simulink model "demonstrator"  (R2021a)
settings: Solver=VariableStepAuto  StartTime=0.0  StopTime=4000/3.2e6  RelTol=1e-3
values from neighbouring files (symbols this model uses):
  f_system = 64e6    (= 64000000)    [setup_demonstrator.m]
  fir_bbuf = reshape([fir_barker_13; fir_barker_13; fir_barker_13], [1, length(fir_barker_13)*3])    [setup_demonstrator.m]
  tx_data = [tx_data mbuf]    [setup_demonstrator.m]
undefined symbols (not defined in the file or in its folder): AXI4, designMultirateFIR, fsystem, Lite, xlfda_numerator
libraries: hdlBasic x533, hdlsllib x35, hdlDSPIP x21, hdlSSR x18, dspmlti4 x14, dspswit3 x8, dspsigops x5, vmcUtilities x4, hdlUtilities x4, simulink x3, dspsigattribs x2, commrandsrc3 x1
(part 5 of 10)

== system demonstrator/Receiver/AXI-Stream Master Interface/Rising Edge Detector Enable ==
  Input : Inport
  Inverter2 : hdlBasic/Inverter  en=off  latency=0  XmcBlockStatus=1  maskContainerNames=group2  block_type=inv  block_config=sysgen:Inverter_config
  Logical3 : hdlBasic/Logical  logical_function=AND  inputs=2  en=off  latency=0  precision=Full  arith_type=Unsigned  n_bits=16  bin_pt=0  align_bp=on  overflow=[]  quantization=[]  XmcBlockStatus=1  maskContainerNames=tabcontainer1  block_type=logical  block_config=sysgen:Logical_config
  Register1 : hdlBasic/Register  init=0  rst=off  en=off  XmcBlockStatus=1  maskContainerNames=tabcontainer1  block_type=register  block_config=sysgen:Register_config
  Output : Outport  VectorParamsAs1DForOutWhenUnconnected=off
  wires:
  Input/1 -> Logical3/2, Inverter2/1
  Inverter2/1 -> Register1/1
  Logical3/1 -> Output/1
  Register1/1 -> Logical3/1

== system demonstrator/Receiver/AXI-Stream Master Interface/Rising Edge Detector Last ==
  Input : Inport
  Inverter2 : hdlBasic/Inverter  en=off  latency=0  XmcBlockStatus=1  maskContainerNames=group2  block_type=inv  block_config=sysgen:Inverter_config
  Logical3 : hdlBasic/Logical  logical_function=AND  inputs=2  en=off  latency=0  precision=Full  arith_type=Unsigned  n_bits=16  bin_pt=0  align_bp=on  overflow=[]  quantization=[]  XmcBlockStatus=1  maskContainerNames=tabcontainer1  block_type=logical  block_config=sysgen:Logical_config
  Register1 : hdlBasic/Register  init=0  rst=off  en=off  XmcBlockStatus=1  maskContainerNames=tabcontainer1  block_type=register  block_config=sysgen:Register_config
  Output : Outport  VectorParamsAs1DForOutWhenUnconnected=off
  wires:
  Register1/1 -> Logical3/1
  Logical3/1 -> Output/1
  Inverter2/1 -> Register1/1
  Input/1 -> Inverter2/1, Logical3/2

== system demonstrator/Receiver/Carrier Synchronisation/De-Rotate Constellation ==
  Imag In : Inport
  Real In : Inport  Port=2
  Valid In : Inport  Port=3
  Imag Error : Inport  Port=4
  Real Error : Inport  Port=5
  Valid Error : Inport  Port=6
  Delay : hdlBasic/Delay  rst=off  en=off  latency=4  reg_retiming=off  XmcBlockStatus=1  maskContainerNames=group1  block_type=delay  block_config=sysgen:Delay_config
  Product : hdlBasic/Product  complex_multiplier=on  optimizegoal=Performance  simulation_type=fast_sim  simulation_model=sysgen:product_macro  XmcBlockStatus=1  maskContainerNames=<empty>  block_type=product_macro  block_config=sysgen:ProductMacro_config
  Register{,1..3} (4 alike) : hdlBasic/Register  init=0  rst=off  en=on  XmcBlockStatus=1  maskContainerNames=tabcontainer1  block_type=register  block_config=sysgen:Register_config
  Register{4..7} (4 alike) : hdlBasic/Register  init=0  rst=off  en=off  XmcBlockStatus=1  maskContainerNames=tabcontainer1  block_type=register  block_config=sysgen:Register_config
  Imag Out : Outport  VectorParamsAs1DForOutWhenUnconnected=off
  Real Out : Outport  Port=2  VectorParamsAs1DForOutWhenUnconnected=off
  Valid Out : Outport  Port=3  VectorParamsAs1DForOutWhenUnconnected=off
  wires:
  Register/1 -> Real Out/1
  Register1/1 -> Imag Out/1
  Valid In/1 -> Register7/1
  Imag Error/1 -> Register3/1
  Register4/1 -> Valid Out/1
  Register7/1 -> Delay/1
  Real Error/1 -> Register2/1
  Imag In/1 -> Register5/1
  Real In/1 -> Register6/1
  Valid Error/1 -> Register3/2, Register2/2
  Delay/1 -> Register/2, Register1/2, Register4/1
  Register6/1 -> Product/1
  Register5/1 -> Product/2
  Register2/1 -> Product/3
  Register3/1 -> Product/4
  Product/1 -> Register/1
  Product/2 -> Register1/1

== system demonstrator/Receiver/Carrier Synchronisation/Generate Angle Error ==
  Imag In : Inport
  Real In : Inport  Port=2
  Valid In : Inport  Port=3
  Circular CORDIC : Subsystem
  Delay : hdlBasic/Delay  rst=off  en=off  latency=8  reg_retiming=off  XmcBlockStatus=1  maskContainerNames=group1  block_type=delay  block_config=sysgen:Delay_config
  Register : hdlBasic/Register  init=0  rst=off  en=on  XmcBlockStatus=1  maskContainerNames=tabcontainer1  block_type=register  block_config=sysgen:Register_config
  Register1 : hdlBasic/Register  init=0  rst=off  en=on  XmcBlockStatus=1  maskContainerNames=tabcontainer1  block_type=register  block_config=sysgen:Register_config
  Register3 : hdlBasic/Register  init=0  rst=off  en=off  XmcBlockStatus=1  maskContainerNames=tabcontainer1  block_type=register  block_config=sysgen:Register_config
  Angle : Outport  VectorParamsAs1DForOutWhenUnconnected=off
  Valid Out : Outport  Port=2  VectorParamsAs1DForOutWhenUnconnected=off
  wires:
  Delay/1 -> Valid Out/1
  Circular CORDIC/1(Angle) -> Angle/1
  Valid In/1 -> Register3/1, Register/2, Register1/2
  Real In/1 -> Register/1
  Imag In/1 -> Register1/1
  Register1/1 -> Circular CORDIC/1(Imag In)
  Register3/1 -> Delay/1
  Register/1 -> Circular CORDIC/2(Real In)

== system demonstrator/Receiver/Carrier Synchronisation/Generate NCO ==
  Angle : Inport
  Valid In : Inport  Port=2
  Reset : Inport  Port=3
  Loop Filter : Subsystem  mask{T=1/(100e3*32), d=0.707, Kp=1, Bn=0.04*(100e3*32), Ko=1}
      mask prompts: T "Sampling Period:"; d "Damping Ratio:"; Kp "Phase Detector Gain:"; Bn "Noise Bandwidth:"; Ko "Oscillator Gain:"
      mask init:
      | n = (Bn*T)/(d+1/(4*d));
      | 
      | %K1 = ((4*d*n)/(1+2*d*n+n^2))/(Ko*Kp);
      | 
      | %K2 = ((4*n^2)/(1+2*d*n+n^2))/(Ko*Kp);
      | 
      | K1 = (4*d*n)/(Ko*Kp);
      | 
      | K2 = (4*(n^2))/(Ko*Kp);
  NCO : Subsystem  mask(NCO){n=8, b=32-8}
      mask prompts: n "Number of integer_bits"; b "Number of fractional bits"
      mask help:
      | Numerically Controller Oscillator.
      |
      | Integrates the phase error and generates cosine and negative sign outputs.
      mask init:
      | k_n = ceil(log2((2^n)/(2*pi)));
      mask DialogControl Container3 Prompt: Accumulator
  Imag Out : Outport  VectorParamsAs1DForOutWhenUnconnected=off
  Real Out : Outport  Port=2  VectorParamsAs1DForOutWhenUnconnected=off
  Valid Out : Outport  Port=3  VectorParamsAs1DForOutWhenUnconnected=off
  wires:
  Reset/1 -> Loop Filter/3(Reset)
  NCO/1(Cos) -> Real Out/1
  NCO/2(Neg Sin) -> Imag Out/1
  Loop Filter/2(Valid) -> NCO/2(En_in)
  Loop Filter/1(Error) -> NCO/1(Step Size)
  Valid In/1 -> Loop Filter/2(Strobe)
  Angle/1 -> Loop Filter/1(Signal)
  NCO/3(En_out) -> Valid Out/1

== system demonstrator/Receiver/Coarse Frequency Synchronisation/Apply Frequency Offset Correction ==
  Imag In : Inport
  Real In : Inport  Port=2
  cos : Inport  Port=3
  sin : Inport  Port=4
  Convert : hdlBasic/Convert  gui_display_data_type=Fixed-point  arith_type=Signed (2's comp)  n_bits=16  bin_pt=14  float_type=Single  exp_bits=8  fraction_bits=24  quantization=Truncate  overflow=Saturate  en=off  latency=0  pipeline=off  XmcBlockStatus=1  maskContainerNames=group2  block_type=convert  block_config=sysgen:Convert_config
  Convert1 : hdlBasic/Convert  gui_display_data_type=Fixed-point  arith_type=Signed (2's comp)  n_bits=16  bin_pt=14  float_type=Single  exp_bits=8  fraction_bits=24  quantization=Truncate  overflow=Saturate  en=off  latency=0  pipeline=off  XmcBlockStatus=1  maskContainerNames=group2  block_type=convert  block_config=sysgen:Convert_config
  Product : hdlBasic/Product  complex_multiplier=on  optimizegoal=Performance  simulation_type=fast_sim  simulation_model=sysgen:product_macro  XmcBlockStatus=1  maskContainerNames=<empty>  block_type=product_macro  block_config=sysgen:ProductMacro_config
  Imag Out : Outport  VectorParamsAs1DForOutWhenUnconnected=off
  Real Out : Outport  Port=2  VectorParamsAs1DForOutWhenUnconnected=off
  wires:
  Product/1 -> Convert/1
  Product/2 -> Convert1/1
  Imag In/1 -> Product/2
  Real In/1 -> Product/1
  cos/1 -> Product/3
  sin/1 -> Product/4
  Convert/1 -> Real Out/1
  Convert1/1 -> Imag Out/1

== system demonstrator/Receiver/Coarse Frequency Synchronisation/Get Frequency Offset ==
  Mag In : Inport
  SoF : Inport  Port=2
  Constant : hdlBasic/Constant  const=1023  gui_display_data_type=Fixed-point  arith_type=Unsigned  n_bits=10  bin_pt=0  preci_type=Single  exp_width=8  frac_width=24  explicit_period=off  period=1  XmcBlockStatus=1  maskContainerNames=tabcontainer1  block_type=constant  block_config=sysgen:Constant_config
  Counter : hdlBasic/Counter  cnt_type=Count limited  cnt_to=1023  operation=Up  start_count=0  cnt_by_val=1  arith_type=Unsigned  n_bits=10  bin_pt=0  load_pin=off  rst=on  en=off  explicit_period=Inferred from inputs  period=1  use_behavioral_HDL=off  implementation=Fabric  XmcBlockStatus=1  maskContainerNames=group1  block_type=counter  block_config=sysgen:Counter_config
  ROM : hdlBasic/ROM  depth=1024  initVector=[0:-1:-1024/2+1, 1024/2:-1:1]*(12.8e6/(1024*4))  distributed_mem=Block RAM  rst=off  init_reg=0  en=off  latency=1  gui_display_data_type=Fixed-point  arith_type="Signed  (2's comp)"  n_bits=32  bin_pt=32-ceil(log2(12.8e6/8))-1  preci_type=Single  exp_width=8  frac_width=24  optimize=Area  use_rpm=on  simulation_type=fast_sim  XmcBlockStatus=1  maskContainerNames=tabcontainer1  block_type=sprom  block_config=sysgen:SPROM_config
  Register : hdlBasic/Register  init=0  rst=off  en=on  XmcBlockStatus=1  maskContainerNames=tabcontainer1  block_type=register  block_config=sysgen:Register_config
  Register1 : hdlBasic/Register  init=0  rst=off  en=on  XmcBlockStatus=1  maskContainerNames=tabcontainer1  block_type=register  block_config=sysgen:Register_config
  Register2 : hdlBasic/Register  init=0  rst=off  en=off  XmcBlockStatus=1  maskContainerNames=tabcontainer1  block_type=register  block_config=sysgen:Register_config
  Register3 : hdlBasic/Register  init=0  rst=off  en=off  XmcBlockStatus=1  maskContainerNames=tabcontainer1  block_type=register  block_config=sysgen:Register_config
  Register4 : hdlBasic/Register  init=0  rst=on  en=on  XmcBlockStatus=1  maskContainerNames=tabcontainer1  block_type=register  block_config=sysgen:Register_config
  Relational : hdlBasic/Relational  mode=a=b  op_type=Bool  en=off  latency=0  XmcBlockStatus=1  maskContainerNames=tabcontainer1  block_type=relational  block_config=sysgen:Relational_config
  Relational2 : hdlBasic/Relational  mode=a>b  op_type=Bool  en=off  latency=0  XmcBlockStatus=1  maskContainerNames=tabcontainer1  block_type=relational  block_config=sysgen:Relational_config
  Offset Out : Outport  VectorParamsAs1DForOutWhenUnconnected=off
  wires:
  Register3/1 -> Register4/1, Relational2/1
  SoF/1 -> Counter/1
  Counter/1 -> Relational/2, Register/1
  Constant/1 -> Relational/1
  Relational/1 -> Register2/1, Register4/2
  Register4/1 -> Relational2/2
  Relational2/1 -> Register/2, Register4/3
  Register/1 -> Register1/1
  Register2/1 -> Register1/2
  Register1/1 -> ROM/1
  ROM/1 -> Offset Out/1
  Mag In/1 -> Register3/1

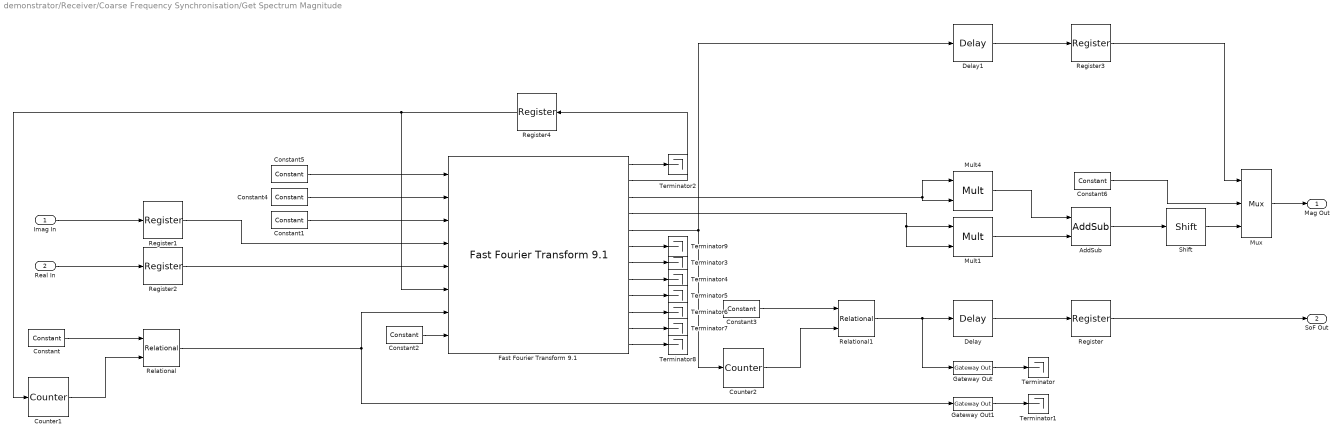
== system demonstrator/Receiver/Coarse Frequency Synchronisation/Get Spectrum Magnitude ==
  Imag In : Inport
  Real In : Inport  Port=2
  AddSub : hdlBasic/AddSub  mode=Addition  use_carryin=off  use_carryout=off  en=off  latency=1  precision=Full  arith_type=Unsigned  n_bits=16  bin_pt=14  quantization=Truncate  overflow=Wrap  use_behavioral_HDL=off  hw_selection=Fabric  pipelined=off  XmcBlockStatus=1  maskContainerNames=tabcontainer1  block_type=addsub  block_config=sysgen:Addsub_config
  Constant : hdlBasic/Constant  const=1023  gui_display_data_type=Fixed-point  arith_type=Unsigned  n_bits=10  bin_pt=0  preci_type=Single  exp_width=8  frac_width=24  explicit_period=on  period=1/12.8e6  XmcBlockStatus=1  maskContainerNames=tabcontainer1  block_type=constant  block_config=sysgen:Constant_config
  Constant1 : hdlBasic/Constant  const=0  gui_display_data_type=Boolean  arith_type=Boolean  n_bits=16  bin_pt=14  preci_type=Single  exp_width=8  frac_width=24  explicit_period=on  period=1/12.8e6  XmcBlockStatus=1  maskContainerNames=tabcontainer1  block_type=constant  block_config=sysgen:Constant_config
  Constant2 : hdlBasic/Constant  const=1  gui_display_data_type=Boolean  arith_type=Boolean  n_bits=16  bin_pt=14  preci_type=Single  exp_width=8  frac_width=24  explicit_period=on  period=1/12.8e6  XmcBlockStatus=1  maskContainerNames=tabcontainer1  block_type=constant  block_config=sysgen:Constant_config
  Constant3 : hdlBasic/Constant  const=0  gui_display_data_type=Fixed-point  arith_type=Unsigned  n_bits=10  bin_pt=0  preci_type=Single  exp_width=8  frac_width=24  explicit_period=on  period=1/12.8e6  XmcBlockStatus=1  maskContainerNames=tabcontainer1  block_type=constant  block_config=sysgen:Constant_config
  Constant4 : hdlBasic/Constant  const=0  gui_display_data_type=Fixed-point  arith_type=Unsigned  n_bits=1  bin_pt=0  preci_type=Single  exp_width=8  frac_width=24  explicit_period=on  period=1/12.8e6  XmcBlockStatus=1  maskContainerNames=tabcontainer1  block_type=constant  block_config=sysgen:Constant_config
  Constant5 : hdlBasic/Constant  const=0  gui_display_data_type=Fixed-point  arith_type=Unsigned  n_bits=10  bin_pt=0  preci_type=Single  exp_width=8  frac_width=24  explicit_period=on  period=1/12.8e6  XmcBlockStatus=1  maskContainerNames=tabcontainer1  block_type=constant  block_config=sysgen:Constant_config
  Constant6 : hdlBasic/Constant  const=0  gui_display_data_type=Fixed-point  arith_type=Unsigned  n_bits=32  bin_pt=31  preci_type=Single  exp_width=8  frac_width=24  explicit_period=on  period=1/12.8e6  XmcBlockStatus=1  maskContainerNames=tabcontainer1  block_type=constant  block_config=sysgen:Constant_config
  Counter1 : hdlBasic/Counter  cnt_type=Count limited  cnt_to=1023  operation=Up  start_count=0  cnt_by_val=1  arith_type=Unsigned  n_bits=10  bin_pt=0  load_pin=off  rst=off  en=on  explicit_period=Explicit  period=1/12.8e6  use_behavioral_HDL=off  implementation=Fabric  XmcBlockStatus=1  maskContainerNames=group1  block_type=counter  block_config=sysgen:Counter_config
  Counter2 : hdlBasic/Counter  cnt_type=Count limited  cnt_to=1023  operation=Up  start_count=0  cnt_by_val=1  arith_type=Unsigned  n_bits=10  bin_pt=0  load_pin=off  rst=off  en=on  explicit_period=Explicit  period=1/12.8e6  use_behavioral_HDL=off  implementation=Fabric  XmcBlockStatus=1  maskContainerNames=group1  block_type=counter  block_config=sysgen:Counter_config
  Delay : hdlBasic/Delay  rst=off  en=off  latency=3  reg_retiming=off  XmcBlockStatus=1  maskContainerNames=group1  block_type=delay  block_config=sysgen:Delay_config
  Delay1 : hdlBasic/Delay  rst=off  en=off  latency=3  reg_retiming=off  XmcBlockStatus=1  maskContainerNames=group1  block_type=delay  block_config=sysgen:Delay_config
  "Fast Fourier Transform 9.1 " : hdlDSPIP/Fast Fourier Transform 9.1   transform_length=1024  target_clock_frequency=128  target_data_throughput=50  implementation_options=pipelined_streaming_io  run_time_configurable_transform_length=off  phase_factor_width=16  scaling_options=scaled  rounding_modes=truncation  aclken=off  aresetn=off  output_ordering=natural_order  cyclic_prefix_insertion=off  throttle_scheme=nonrealtime  xk_index=off  ovflo=off  trim_axipin_name=on  memory_options_data=block_ram  memory_options_phase_factors=block_ram  number_of_stages_using_block_ram_for_data_and_phase_factors=1  memory_options_reorder=block_ram  memory_options_hybrid=off  complex_mult_type=use_mults_resources  butterfly_type=use_luts  simulation_type=hybrid_sim  simulation_model=sysgen:xfftv9_cmodel  data_path_portlist={ 's_axis_data_tdata', 'm_axis_data_tdata', 'm_axis_status_tdata', 'event_fft_overflow' }  channels=1  input_ordering=natural_order  input_width=16  ip_name=Fast Fourier Transform  ip_version=9.1  dsptool_ready=true  ipcore_usecache=true  ipcore_useipmodelcache=true  wrapper_available=true  port_translation_map={ 'aclken' => 'en', 'aresetn' => 'rst'}  data_format=fixed_point  XmcBlockStatus=1  maskContainerNames=tabcontainer1  block_type=xfft_v9_1  block_config=sysgen:rodinimport_config
  Gateway Out : hdlBasic/Gateway Out  inherit_from_input=on  hdl_port=off  rows=1  columns=1  UseAsDAC=off  DACChannel='1'  interface=None  automatic_assignment=on  address_offset=hex2dec('00')  intf_name=''  intf_description=''  timing_constraint=None  locs_specified=off  LOCs={}  io_standard={}  XmcBlockStatus=1  maskContainerNames=group4  block_type=gatewayout  block_config=sysgen:gateway_out_config  block_width_w=590  block_height_w=620  block_width=620  block_height=750
  Gateway Out1 : hdlBasic/Gateway Out  inherit_from_input=on  hdl_port=off  rows=1  columns=1  UseAsDAC=off  DACChannel='1'  interface=None  automatic_assignment=on  address_offset=hex2dec('00')  intf_name=''  intf_description=''  timing_constraint=None  locs_specified=off  LOCs={}  io_standard={}  XmcBlockStatus=1  maskContainerNames=group4  block_type=gatewayout  block_config=sysgen:gateway_out_config  block_width_w=590  block_height_w=620  block_width=620  block_height=750
  Mult1 : hdlBasic/Mult  precision=User Defined  arith_type=Unsigned  n_bits=63  bin_pt=62  quantization=Truncate  overflow=Saturate  en=off  latency=3  use_behavioral_HDL=off  opt=Speed  use_embedded=on  optimum_pipeline=off  pipeline=on  use_rpm=on  placement_style=Triangular  XmcBlockStatus=1  maskContainerNames=group1  block_type=mult  block_config=sysgen:Mult_config
  Mult4 : hdlBasic/Mult  precision=User Defined  arith_type=Unsigned  n_bits=63  bin_pt=62  quantization=Truncate  overflow=Saturate  en=off  latency=3  use_behavioral_HDL=off  opt=Speed  use_embedded=on  optimum_pipeline=off  pipeline=on  use_rpm=on  placement_style=Triangular  XmcBlockStatus=1  maskContainerNames=group1  block_type=mult  block_config=sysgen:Mult_config
  Mux : hdlBasic/Mux  inputs=2  en=off  latency=0  precision=Full  arith_type=Unsigned  n_bits=16  bin_pt=14  quantization=Truncate  overflow=Wrap  XmcBlockStatus=1  maskContainerNames=tabcontainer1  block_type=mux  block_config=sysgen:Mux_config
  Register{,1..4} (5 alike) : hdlBasic/Register  init=0  rst=off  en=off  XmcBlockStatus=1  maskContainerNames=tabcontainer1  block_type=register  block_config=sysgen:Register_config
  Relational : hdlBasic/Relational  mode=a=b  op_type=Bool  en=off  latency=0  XmcBlockStatus=1  maskContainerNames=tabcontainer1  block_type=relational  block_config=sysgen:Relational_config
  Relational1 : hdlBasic/Relational  mode=a=b  op_type=Bool  en=off  latency=0  XmcBlockStatus=1  maskContainerNames=tabcontainer1  block_type=relational  block_config=sysgen:Relational_config
  Shift : hdlBasic/Shift  shift_dir=Right  shift_bits=2  en=off  latency=0  precision=User Defined  arith_type=Unsigned  n_bits=32  bin_pt=31  quantization=Truncate  overflow=Wrap  XmcBlockStatus=1  maskContainerNames=group2  block_type=shift  block_config=sysgen:Shift_config
  Terminator{,1..9} (10 alike) : Terminator
  Mag Out : Outport  VectorParamsAs1DForOutWhenUnconnected=off
  SoF Out : Outport  Port=2  VectorParamsAs1DForOutWhenUnconnected=off
  wires:
  Register3/1 -> Mux/1
  Delay1/1 -> Register3/1
  Constant6/1 -> Mux/2
  Shift/1 -> Mux/3
  Mux/1 -> Mag Out/1
  Constant5/1 -> "Fast Fourier Transform 9.1 "/1
  Constant4/1 -> "Fast Fourier Transform 9.1 "/2
  "Fast Fourier Transform 9.1 "/6 -> Terminator9/1
  "Fast Fourier Transform 9.1 "/5 -> Delay1/1, Counter2/1
  Constant3/1 -> Relational1/1
  Counter2/1 -> Relational1/2
  "Fast Fourier Transform 9.1 "/12 -> Terminator8/1
  "Fast Fourier Transform 9.1 "/11 -> Terminator7/1
  "Fast Fourier Transform 9.1 "/10 -> Terminator6/1
  "Fast Fourier Transform 9.1 "/9 -> Terminator5/1
  "Fast Fourier Transform 9.1 "/8 -> Terminator4/1
  "Fast Fourier Transform 9.1 "/7 -> Terminator3/1
  Constant1/1 -> "Fast Fourier Transform 9.1 "/3
  "Fast Fourier Transform 9.1 "/1 -> Terminator2/1
  Counter1/1 -> Relational/2
  Gateway Out1/1 -> Terminator1/1
  Gateway Out/1 -> Terminator/1
  Relational/1 -> Gateway Out1/1, "Fast Fourier Transform 9.1 "/7
  Constant/1 -> Relational/1
  Relational1/1 -> Delay/1, Gateway Out/1
  "Fast Fourier Transform 9.1 "/4 -> Mult1/2, Mult1/1
  Real In/1 -> Register2/1
  "Fast Fourier Transform 9.1 "/3 -> Mult4/2, Mult4/1
  Imag In/1 -> Register1/1
  Delay/1 -> Register/1
  Register/1 -> SoF Out/1
  Register1/1 -> "Fast Fourier Transform 9.1 "/4
  Register2/1 -> "Fast Fourier Transform 9.1 "/5
  Mult1/1 -> AddSub/2
  Mult4/1 -> AddSub/1
  AddSub/1 -> Shift/1
  Register4/1 -> Counter1/1, "Fast Fourier Transform 9.1 "/6
  "Fast Fourier Transform 9.1 "/2 -> Register4/1
  Constant2/1 -> "Fast Fourier Transform 9.1 "/8

== system demonstrator/Receiver/Coarse Frequency Synchronisation/Increase Signal Power ==
  note: 18-bit multiply for DSP48E2
  note: Product block is required as it is a complex multiplication
  Imag In : Inport
  Real In : Inport  Port=2
  Convert : hdlBasic/Convert  gui_display_data_type=Fixed-point  arith_type=Signed (2's comp)  n_bits=32  bin_pt=31  float_type=Single  exp_bits=8  fraction_bits=24  quantization=Truncate  overflow=Wrap  en=off  latency=0  pipeline=off  XmcBlockStatus=1  maskContainerNames=group2  block_type=convert  block_config=sysgen:Convert_config
  Convert1 : hdlBasic/Convert  gui_display_data_type=Fixed-point  arith_type=Signed (2's comp)  n_bits=32  bin_pt=31  float_type=Single  exp_bits=8  fraction_bits=24  quantization=Truncate  overflow=Wrap  en=off  latency=0  pipeline=off  XmcBlockStatus=1  maskContainerNames=group2  block_type=convert  block_config=sysgen:Convert_config
  Convert2 : hdlBasic/Convert  gui_display_data_type=Fixed-point  arith_type=Signed (2's comp)  n_bits=18  bin_pt=15  float_type=Single  exp_bits=8  fraction_bits=24  quantization=Truncate  overflow=Wrap  en=off  latency=0  pipeline=off  XmcBlockStatus=1  maskContainerNames=group2  block_type=convert  block_config=sysgen:Convert_config
  Convert4 : hdlBasic/Convert  gui_display_data_type=Fixed-point  arith_type=Signed (2's comp)  n_bits=18  bin_pt=15  float_type=Single  exp_bits=8  fraction_bits=24  quantization=Truncate  overflow=Wrap  en=off  latency=0  pipeline=off  XmcBlockStatus=1  maskContainerNames=group2  block_type=convert  block_config=sysgen:Convert_config
  Product1 : hdlBasic/Product  complex_multiplier=on  optimizegoal=Performance  simulation_type=fast_sim  simulation_model=sysgen:product_macro  XmcBlockStatus=1  maskContainerNames=<empty>  block_type=product_macro  block_config=sysgen:ProductMacro_config
  Product2 : hdlBasic/Product  complex_multiplier=on  optimizegoal=Performance  simulation_type=fast_sim  simulation_model=sysgen:product_macro  XmcBlockStatus=1  maskContainerNames=<empty>  block_type=product_macro  block_config=sysgen:ProductMacro_config
  Imag Out : Outport  VectorParamsAs1DForOutWhenUnconnected=off
  Real Out : Outport  Port=2  VectorParamsAs1DForOutWhenUnconnected=off
  wires:
  Imag In/1 -> Product2/2, Product2/4
  Real In/1 -> Product2/1, Product2/3
  Product2/1 -> Convert4/1
  Product2/2 -> Convert2/1
  Convert4/1 -> Product1/1, Product1/3
  Convert2/1 -> Product1/4, Product1/2
  Product1/1 -> Convert/1
  Product1/2 -> Convert1/1
  Convert/1 -> Real Out/1
  Convert1/1 -> Imag Out/1

== system demonstrator/Receiver/Coarse Frequency Synchronisation/NCO ==
  Offset In : Inport
  AddSub : hdlBasic/AddSub  mode=Addition  use_carryin=off  use_carryout=off  en=off  latency=0  precision=User Defined  arith_type=Unsigned  n_bits=41  bin_pt=41-10  quantization=Truncate  overflow=Wrap  use_behavioral_HDL=off  hw_selection=Fabric  pipelined=off  XmcBlockStatus=1  maskContainerNames=tabcontainer1  block_type=addsub  block_config=sysgen:Addsub_config
  CMult : hdlBasic/CMult  const=1024/(12.8e6)  gui_display_data_type=Fixed-point  const_n_bits=i+b  const_bin_pt=b  float_type=Single  exp_bits=8  fraction_bits=24  en=off  latency=1  precision=User Defined  arith_type="Signed  (2's comp)"  n_bits=n+b  bin_pt=b  quantization=Truncate  overflow=Saturate  use_behavioral_HDL=off  mem_type=Distributed RAM  pipeline=off  XmcBlockStatus=1  maskContainerNames=tabcontainer1  block_type=cmult  block_config=sysgen:CMult_config
      settings: infoedit=[]
  Convert4 : hdlBasic/Convert  gui_display_data_type=Fixed-point  arith_type=Unsigned  n_bits=10  bin_pt=0  float_type=Single  exp_bits=8  fraction_bits=24  quantization=Truncate  overflow=Wrap  en=off  latency=0  pipeline=off  XmcBlockStatus=1  maskContainerNames=group2  block_type=convert  block_config=sysgen:Convert_config
  Delay2 : hdlBasic/Delay  rst=off  en=off  latency=1  reg_retiming=off  XmcBlockStatus=1  maskContainerNames=group1  block_type=delay  block_config=sysgen:Delay_config
  Sin_ROM : hdlBasic/ROM  depth=1024  initVector=sin(pi*(0:1024-1)/(1024/2))  distributed_mem=Block RAM  rst=off  init_reg=0  en=off  latency=1  gui_display_data_type=Fixed-point  arith_type="Signed  (2's comp)"  n_bits=L  bin_pt=L-2  preci_type=Single  exp_width=8  frac_width=24  optimize=Area  use_rpm=on  simulation_type=fast_sim  XmcBlockStatus=1  maskContainerNames=tabcontainer1  block_type=sprom  block_config=sysgen:SPROM_config
  cos_ROM : hdlBasic/ROM  depth=1024  initVector=cos(pi*(0:1024-1)/(1024/2))  distributed_mem=Block RAM  rst=off  init_reg=0  en=off  latency=1  gui_display_data_type=Fixed-point  arith_type="Signed  (2's comp)"  n_bits=L  bin_pt=L-2  preci_type=Single  exp_width=8  frac_width=24  optimize=Area  use_rpm=on  simulation_type=fast_sim  XmcBlockStatus=1  maskContainerNames=tabcontainer1  block_type=sprom  block_config=sysgen:SPROM_config
  cos : Outport  VectorParamsAs1DForOutWhenUnconnected=off
  sin : Outport  Port=2  VectorParamsAs1DForOutWhenUnconnected=off
  wires:
  cos_ROM/1 -> cos/1
  Sin_ROM/1 -> sin/1
  Convert4/1 -> cos_ROM/1, Sin_ROM/1
  CMult/1 -> AddSub/2
  Delay2/1 -> AddSub/1
  Offset In/1 -> CMult/1
  AddSub/1 -> Delay2/1, Convert4/1

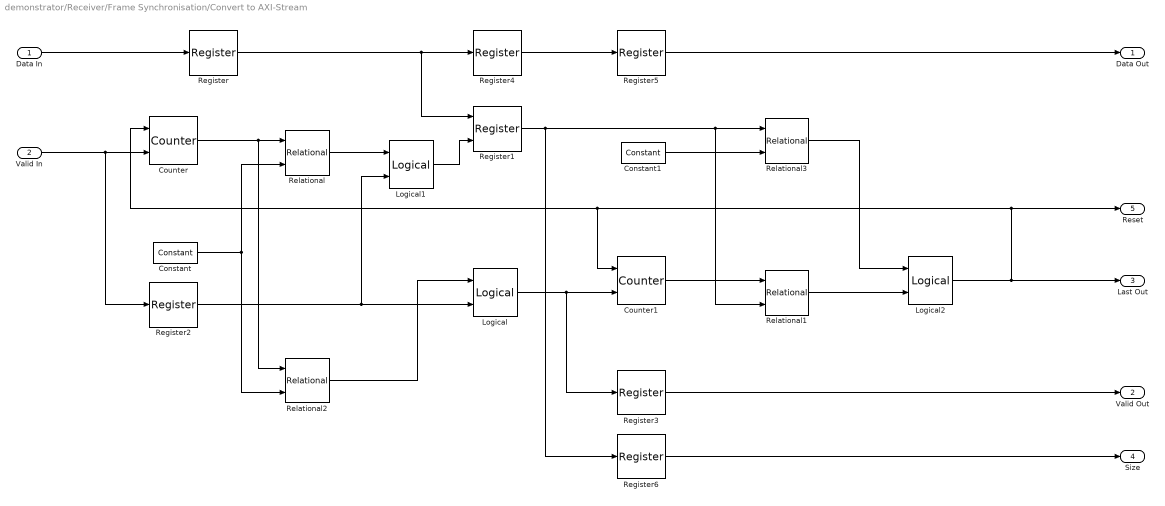
== system demonstrator/Receiver/Frame Synchronisation/Convert to AXI-Stream ==
  Data In : Inport
  Valid In : Inport  Port=2
  Constant : hdlBasic/Constant  const=1.0  gui_display_data_type=Fixed-point  arith_type=Unsigned  n_bits=1  bin_pt=0  preci_type=Single  exp_width=8  frac_width=24  explicit_period=off  period=1  XmcBlockStatus=1  maskContainerNames=tabcontainer1  block_type=constant  block_config=sysgen:Constant_config
  Constant1 : hdlBasic/Constant  const=0  gui_display_data_type=Fixed-point  arith_type=Unsigned  n_bits=1  bin_pt=0  preci_type=Single  exp_width=8  frac_width=24  explicit_period=off  period=1  XmcBlockStatus=1  maskContainerNames=tabcontainer1  block_type=constant  block_config=sysgen:Constant_config
  Counter : hdlBasic/Counter  cnt_type=Free running  cnt_to=Inf  operation=Up  start_count=0  cnt_by_val=1  arith_type=Unsigned  n_bits=32  bin_pt=0  load_pin=off  rst=on  en=on  explicit_period=Inferred from inputs  period=1  use_behavioral_HDL=off  implementation=Fabric  XmcBlockStatus=1  maskContainerNames=group1  block_type=counter  block_config=sysgen:Counter_config
  Counter1 : hdlBasic/Counter  cnt_type=Free running  cnt_to=Inf  operation=Up  start_count=0  cnt_by_val=1  arith_type=Unsigned  n_bits=32  bin_pt=0  load_pin=off  rst=on  en=on  explicit_period=Inferred from inputs  period=1  use_behavioral_HDL=off  implementation=Fabric  XmcBlockStatus=1  maskContainerNames=group1  block_type=counter  block_config=sysgen:Counter_config
  Logical : hdlBasic/Logical  logical_function=AND  inputs=2  en=off  latency=1  precision=Full  arith_type=Unsigned  n_bits=16  bin_pt=0  align_bp=on  overflow=[]  quantization=[]  XmcBlockStatus=1  maskContainerNames=tabcontainer1  block_type=logical  block_config=sysgen:Logical_config
  Logical1 : hdlBasic/Logical  logical_function=AND  inputs=2  en=off  latency=0  precision=Full  arith_type=Unsigned  n_bits=16  bin_pt=0  align_bp=on  overflow=[]  quantization=[]  XmcBlockStatus=1  maskContainerNames=tabcontainer1  block_type=logical  block_config=sysgen:Logical_config
  Logical2 : hdlBasic/Logical  logical_function=AND  inputs=2  en=off  latency=0  precision=Full  arith_type=Unsigned  n_bits=16  bin_pt=0  align_bp=on  overflow=[]  quantization=[]  XmcBlockStatus=1  maskContainerNames=tabcontainer1  block_type=logical  block_config=sysgen:Logical_config
  Register{,2..6} (6 alike) : hdlBasic/Register  init=0  rst=off  en=off  XmcBlockStatus=1  maskContainerNames=tabcontainer1  block_type=register  block_config=sysgen:Register_config
  Register1 : hdlBasic/Register  init=0  rst=off  en=on  XmcBlockStatus=1  maskContainerNames=tabcontainer1  block_type=register  block_config=sysgen:Register_config
  Relational : hdlBasic/Relational  mode=a=b  op_type=Bool  en=off  latency=0  XmcBlockStatus=1  maskContainerNames=tabcontainer1  block_type=relational  block_config=sysgen:Relational_config
  Relational1 : hdlBasic/Relational  mode=a>=b  op_type=Bool  en=off  latency=0  XmcBlockStatus=1  maskContainerNames=tabcontainer1  block_type=relational  block_config=sysgen:Relational_config
  Relational2 : hdlBasic/Relational  mode=a>b  op_type=Bool  en=off  latency=0  XmcBlockStatus=1  maskContainerNames=tabcontainer1  block_type=relational  block_config=sysgen:Relational_config
  Relational3 : hdlBasic/Relational  mode=a!=b  op_type=Bool  en=off  latency=0  XmcBlockStatus=1  maskContainerNames=tabcontainer1  block_type=relational  block_config=sysgen:Relational_config
  Data Out : Outport  VectorParamsAs1DForOutWhenUnconnected=off
  Valid Out : Outport  Port=2  VectorParamsAs1DForOutWhenUnconnected=off
  Last Out : Outport  Port=3  VectorParamsAs1DForOutWhenUnconnected=off
  Size : Outport  Port=4  VectorParamsAs1DForOutWhenUnconnected=off
  Reset : Outport  Port=5  VectorParamsAs1DForOutWhenUnconnected=off
  wires:
  Register6/1 -> Size/1
  Logical2/1 -> Last Out/1, Reset/1, Counter1/1, Counter/1
  Relational1/1 -> Logical2/2
  Relational3/1 -> Logical2/1
  Constant1/1 -> Relational3/2
  Logical1/1 -> Register1/2
  Relational/1 -> Logical1/1
  Relational2/1 -> Logical/1
  Constant/1 -> Relational2/2, Relational/2
  Register5/1 -> Data Out/1
  Register4/1 -> Register5/1
  Register3/1 -> Valid Out/1
  Register2/1 -> Logical/2, Logical1/2
  Register1/1 -> Relational1/2, Relational3/1, Register6/1
  Counter1/1 -> Relational1/1
  Logical/1 -> Counter1/2, Register3/1
  Register/1 -> Register1/1, Register4/1
  Data In/1 -> Register/1
  Counter/1 -> Relational/1, Relational2/1
  Valid In/1 -> Counter/2, Register2/1

== system demonstrator/Receiver/Frame Synchronisation/Frame Sync ==
  Threshold : Inport
  Data In : Inport  Port=2
  Valid In : Inport  Port=3
  reset_count : Inport  Port=4
  Reset : Inport  Port=5
  Counter1 : hdlBasic/Counter  cnt_type=Free running  cnt_to=Inf  operation=Up  start_count=0  cnt_by_val=1  arith_type=Unsigned  n_bits=32  bin_pt=0  load_pin=off  rst=on  en=on  explicit_period=Inferred from inputs  period=1  use_behavioral_HDL=off  implementation=Fabric  XmcBlockStatus=1  maskContainerNames=group1  block_type=counter  block_config=sysgen:Counter_config
  DBPSK Convert : Subsystem
  DBPSK Decision : Subsystem
  Delay : hdlBasic/Delay  rst=off  en=off  latency=2  reg_retiming=off  XmcBlockStatus=1  maskContainerNames=group1  block_type=delay  block_config=sysgen:Delay_config
  Delay1 : hdlBasic/Delay  rst=off  en=on  latency=2  reg_retiming=off  XmcBlockStatus=1  maskContainerNames=group1  block_type=delay  block_config=sysgen:Delay_config
  "FIR Compiler 7.2 " : hdlDSPIP/FIR Compiler 7.2   coefficientvector=fliplr(double(fir_bbuf))  coefficient_sets=1  coefficient_reload=off  filter_type=Single_Rate  rate_change_type=Integer  interpolation_rate=1  decimation_rate=1  zero_pack_factor=1  channel_sequence=Basic  number_channels=1  pattern_list='P4-0,P4-1,P4-2,P4-3,P4-4'  number_paths=1  ratespecification=Maximum_Possible  sampleperiod=0.50000000  hardwareoversamplingrate=1  coefficient_sign=Signed  quantization=Integer_Coefficients  coefficient_width=2  bestprecision=off  coefficient_fractional_bits=0  coefficient_structure=Inferred  output_rounding_mode=Full_Precision  output_width=22  filter_architecture=Systolic_Multiply_Accumulate  optimization_goal=Area  optimization_list='None'  data_buffer_type=Automatic  coefficient_buffer_type=Automatic  input_buffer_type=Automatic  output_buffer_type=Automatic  preference_for_other_storage=Automatic  multi_column_support=Automatic  columnconfig='39'  inter_column_pipe_length=4  data_has_tlast=Not_Required  m_data_has_tready=off  s_data_has_fifo=off  s_data_has_tuser=Not_Required  m_data_has_tuser=Not_Required  s_config_sync_mode=On_Vector  s_config_method=Single  num_reload_slots=1  has_aclken=on  has_aresetn=off  reset_data_vector=on  trim_axipin_name=on  simulation_type=hybrid_sim  simulation_model=sysgen:xfirv7_2_cmodel  data_path_portlist={ 's_axis_data_tdata', 'm_axis_data_tdata' }  passband_min=0.0  passband_max=0.5  stopband_min=0.5  stopband_max=1.0  filter_selection=1  gui_behaviour='Sysgen_GUI'  data_sign=Signed  data_width=16  data_fractional_bits=0  data_tuser_width=1  wrapper_available=true  ip_wrap_arbitrary_binary_point=true  ip_name=FIR Compiler  ip_version=7.2  dsptool_ready=true  ipcore_usecache=true  ipcore_useipmodelcache=true  port_translation_map={ 'aclken' => 'en', 'aresetn' => 'rst' }  run_core_at_system_period=true  ipcore_xco_need_fpga_part=true  ipcore_fpga_part=[]  XmcBlockStatus=1  maskContainerNames=tabcontainer1  block_type=fir_compiler_v7_2  block_config=sysgen:rodinimport_config  block_width=820  block_height=600
  Logical : hdlBasic/Logical  logical_function=AND  inputs=2  en=off  latency=0  precision=Full  arith_type=Unsigned  n_bits=16  bin_pt=0  align_bp=on  overflow=[]  quantization=[]  XmcBlockStatus=1  maskContainerNames=tabcontainer1  block_type=logical  block_config=sysgen:Logical_config
  Logical1 : hdlBasic/Logical  logical_function=OR  inputs=2  en=off  latency=0  precision=Full  arith_type=Unsigned  n_bits=16  bin_pt=0  align_bp=on  overflow=[]  quantization=[]  XmcBlockStatus=1  maskContainerNames=tabcontainer1  block_type=logical  block_config=sysgen:Logical_config
  Register1 : hdlBasic/Register  init=0  rst=on  en=on  XmcBlockStatus=1  maskContainerNames=tabcontainer1  block_type=register  block_config=sysgen:Register_config
  Relational1 : hdlBasic/Relational  mode=a>=b  op_type=Bool  en=off  latency=0  XmcBlockStatus=1  maskContainerNames=tabcontainer1  block_type=relational  block_config=sysgen:Relational_config
  Rising Edge Detector : Subsystem
  Shift Register : Subsystem
  Slice : hdlBasic/Slice  nbits=1  boolean_output=off  mode=Upper Bit Location + Width  bit1=0  base1=MSB of Input  bit0=0  base0=LSB of Input  XmcBlockStatus=1  maskContainerNames=group1  block_type=slice  block_config=sysgen:Slice_config
  Terminator : Terminator
  Terminator1 : Terminator
  Data Out : Outport  VectorParamsAs1DForOutWhenUnconnected=off
  Valid Out : Outport  Port=2  VectorParamsAs1DForOutWhenUnconnected=off
  count : Outport  Port=3  VectorParamsAs1DForOutWhenUnconnected=off
  wires:
  Shift Register/2(Valid Out) -> Valid Out/1
  Data In/1 -> Slice/1
  Delay/1 -> Logical/1
  "FIR Compiler 7.2 "/3 -> Relational1/1
  reset_count/1 -> Counter1/1, Logical1/1
  "FIR Compiler 7.2 "/1 -> Terminator/1
  DBPSK Convert/2(Valid Out) -> "FIR Compiler 7.2 "/2
  Shift Register/1(Data Out) -> Data Out/1
  Register1/1 -> Logical/2
  Rising Edge Detector/1(Output) -> Register1/1, Register1/3, Counter1/2
  "FIR Compiler 7.2 "/2 -> Terminator1/1
  Slice/1 -> DBPSK Decision/1(Data In)
  Valid In/1 -> DBPSK Decision/2(Valid In)
  Counter1/1 -> count/1
  Logical1/1 -> Register1/2
  Threshold/1 -> Relational1/2
  Logical/1 -> Shift Register/2(Valid In)
  Delay1/1 -> Shift Register/1(Data In)
  DBPSK Decision/1(Data Out) -> DBPSK Convert/1(Data In), Delay1/1
  Relational1/1 -> Rising Edge Detector/1(Input)
  Reset/1 -> Logical1/2
  DBPSK Decision/2(Valid Out) -> DBPSK Convert/2(Valid In), Delay/1, Delay1/2
  DBPSK Convert/1(Data Out) -> "FIR Compiler 7.2 "/1

== system demonstrator/Receiver/Observation Point/op ==
  Data In : Inport
  Valid In : Inport  Port=2
  Cast To Boolean : DataTypeConversion  OutDataTypeStr=boolean
  Constellation Diagram : ConstellationDiagram
  Convert Protect : DataTypeConversion  OutDataTypeStr=fixdt(0,32,0)  ConvertRealWorld=Stored Integer (SI)
  Delay : Delay  DelayLength=1  ShowEnablePort=on
      settings: InputPortMap=u0,e6
  Imag Conversion : DataTypeConversion  OutDataTypeStr=fixdt(1,16,15)  ConvertRealWorld=Stored Integer (SI)
  Imag Slice : hdlsllib/Logic and Bit Operations/Bit Slice  lidx=31  ridx=16
      settings: SourceProductBaseCode=SL
  Real Conversion : DataTypeConversion  OutDataTypeStr=fixdt(1,16,15)  ConvertRealWorld=Stored Integer (SI)
  Real Slice : hdlsllib/Logic and Bit Operations/Bit Slice  lidx=15  ridx=0
      settings: SourceProductBaseCode=SL
  Real-Imag to Complex : RealImagToComplex
  Time Scope : Scope
  m_axis_op_tdata : hdlBasic/Gateway Out  inherit_from_input=on  hdl_port=on  rows=1  columns=1  UseAsDAC=off  DACChannel='1'  interface=None  automatic_assignment=on  address_offset=hex2dec('00')  intf_name=''  intf_description=''  timing_constraint=None  locs_specified=off  LOCs={}  io_standard={}  XmcBlockStatus=1  maskContainerNames=group4  block_type=gatewayout  block_config=sysgen:gateway_out_config  block_width_w=590  block_height_w=620  block_width=620  block_height=750
  m_axis_op_tvalid : hdlBasic/Gateway Out  inherit_from_input=on  hdl_port=on  rows=1  columns=1  UseAsDAC=off  DACChannel='1'  interface=None  automatic_assignment=on  address_offset=hex2dec('00')  intf_name=''  intf_description=''  timing_constraint=None  locs_specified=off  LOCs={}  io_standard={}  XmcBlockStatus=1  maskContainerNames=group4  block_type=gatewayout  block_config=sysgen:gateway_out_config  block_width_w=590  block_height_w=620  block_width=620  block_height=750
  wires:
  Cast To Boolean/1 -> Delay/2
  Convert Protect/1 -> Imag Slice/1, Real Slice/1
  Real-Imag to Complex/1 -> Delay/1
  m_axis_op_tdata/1 -> Convert Protect/1
  Imag Conversion/1 -> Real-Imag to Complex/2
  Imag Slice/1 -> Imag Conversion/1
  Real Slice/1 -> Real Conversion/1
  Real Conversion/1 -> Real-Imag to Complex/1
  m_axis_op_tvalid/1 -> Cast To Boolean/1
  Delay/1 -> Constellation Diagram/1, Time Scope/1
  Data In/1 -> m_axis_op_tdata/1
  Valid In/1 -> m_axis_op_tvalid/1

== system demonstrator/Receiver/Time Synchronisation/Loop Filter ==
  note: Get centre of symbol
  note: The input to the loop filter should only be changed once per symbol.
      |
      | Use an enable register with the strobe from the NCC to hold the data in place.
  note: Get centre of symbol
  Real In : Inport
  Imag In : Inport  Port=2
  Signal In : Inport  Port=3
  Valid In : Inport  Port=4
  Reset : Inport  Port=5
  AddSub : hdlBasic/AddSub  mode=Addition  use_carryin=off  use_carryout=off  en=off  latency=0  precision=User Defined  arith_type="Signed  (2's comp)"  n_bits=64  bin_pt=60  quantization=Truncate  overflow=Saturate  use_behavioral_HDL=off  hw_selection=Fabric  pipelined=off  XmcBlockStatus=1  maskContainerNames=tabcontainer1  block_type=addsub  block_config=sysgen:Addsub_config
  AddSub1 : hdlBasic/AddSub  mode=Addition  use_carryin=off  use_carryout=off  en=off  latency=0  precision=User Defined  arith_type="Signed  (2's comp)"  n_bits=64  bin_pt=60  quantization=Truncate  overflow=Saturate  use_behavioral_HDL=off  hw_selection=Fabric  pipelined=off  XmcBlockStatus=1  maskContainerNames=tabcontainer1  block_type=addsub  block_config=sysgen:Addsub_config
  Delay1 : hdlBasic/Delay  rst=off  en=off  latency=32/2  reg_retiming=off  XmcBlockStatus=1  maskContainerNames=group1  block_type=delay  block_config=sysgen:Delay_config
  Delay2 : hdlBasic/Delay  rst=off  en=off  latency=32/2  reg_retiming=off  XmcBlockStatus=1  maskContainerNames=group1  block_type=delay  block_config=sysgen:Delay_config
  Delay3 : hdlBasic/Delay  rst=off  en=off  latency=32/2  reg_retiming=off  XmcBlockStatus=1  maskContainerNames=group1  block_type=delay  block_config=sysgen:Delay_config
  K1_Gain : hdlBasic/CMult  const=K1  gui_display_data_type=Fixed-point  const_n_bits=32  const_bin_pt=30  float_type=Single  exp_bits=8  fraction_bits=24  en=off  latency=0  precision=Full  arith_type="Signed  (2's comp)"  n_bits=3+28+16  bin_pt=28+16  quantization=Truncate  overflow=Wrap  use_behavioral_HDL=off  mem_type=Distributed RAM  pipeline=off  XmcBlockStatus=1  maskContainerNames=tabcontainer1  block_type=cmult  block_config=sysgen:CMult_config
      settings: infoedit=[]
  K2_Gain : hdlBasic/CMult  const=K2  gui_display_data_type=Fixed-point  const_n_bits=32  const_bin_pt=30  float_type=Single  exp_bits=8  fraction_bits=24  en=off  latency=0  precision=Full  arith_type="Signed  (2's comp)"  n_bits=3+28+16  bin_pt=28+16  quantization=Truncate  overflow=Wrap  use_behavioral_HDL=off  mem_type=Distributed RAM  pipeline=off  XmcBlockStatus=1  maskContainerNames=tabcontainer1  block_type=cmult  block_config=sysgen:CMult_config
      settings: infoedit=[]
  Register : hdlBasic/Register  init=0  rst=on  en=on  XmcBlockStatus=1  maskContainerNames=tabcontainer1  block_type=register  block_config=sysgen:Register_config
  Register1 : hdlBasic/Register  init=0  rst=on  en=on  XmcBlockStatus=1  maskContainerNames=tabcontainer1  block_type=register  block_config=sysgen:Register_config
  Real Out : Outport  VectorParamsAs1DForOutWhenUnconnected=off
  Imag Out : Outport  Port=2  VectorParamsAs1DForOutWhenUnconnected=off
  Valid Out : Outport  Port=3  VectorParamsAs1DForOutWhenUnconnected=off
  Error Out : Outport  Port=4  VectorParamsAs1DForOutWhenUnconnected=off
  wires:
  AddSub1/1 -> Error Out/1
  Valid In/1 -> Register1/3, Delay3/1, Register/3
  Delay1/1 -> Real Out/1
  Delay2/1 -> Imag Out/1
  Register1/1 -> K2_Gain/1, K1_Gain/1
  Signal In/1 -> Register1/1
  Register/1 -> AddSub/2
  K1_Gain/1 -> AddSub1/1
  AddSub/1 -> AddSub1/2, Register/1
  Imag In/1 -> Delay2/1
  Real In/1 -> Delay1/1
  K2_Gain/1 -> AddSub/1
  Reset/1 -> Register1/2, Register/2
  Delay3/1 -> Valid Out/1

== system demonstrator/Receiver/Time Synchronisation/NCC ==
  Error : Inport
  AddSub : hdlBasic/AddSub  mode=Addition  use_carryin=off  use_carryout=off  en=off  latency=0  precision=User Defined  arith_type=Unsigned  n_bits=n+f  bin_pt=f  quantization=Truncate  overflow=Wrap  use_behavioral_HDL=off  hw_selection=Fabric  pipelined=off  XmcBlockStatus=1  maskContainerNames=tabcontainer1  block_type=addsub  block_config=sysgen:Addsub_config
  AddSub1 : hdlBasic/AddSub  mode=Addition  use_carryin=off  use_carryout=off  en=off  latency=0  precision=User Defined  arith_type="Signed  (2's comp)"  n_bits=n+f  bin_pt=f  quantization=Truncate  overflow=Saturate  use_behavioral_HDL=off  hw_selection=Fabric  pipelined=off  XmcBlockStatus=1  maskContainerNames=tabcontainer1  block_type=addsub  block_config=sysgen:Addsub_config
  AddSub2 : hdlBasic/AddSub  mode=Subtraction  use_carryin=off  use_carryout=off  en=off  latency=0  precision=User Defined  arith_type="Signed  (2's comp)"  n_bits=n+f  bin_pt=f  quantization=Truncate  overflow=Flag as error  use_behavioral_HDL=off  hw_selection=Fabric  pipelined=off  XmcBlockStatus=1  maskContainerNames=tabcontainer1  block_type=addsub  block_config=sysgen:Addsub_config
  Constant : hdlBasic/Constant  const=1  gui_display_data_type=Fixed-point  arith_type=Unsigned  n_bits=1  bin_pt=0  preci_type=Single  exp_width=8  frac_width=24  explicit_period=off  period=1  XmcBlockStatus=1  maskContainerNames=tabcontainer1  block_type=constant  block_config=sysgen:Constant_config
  Constant1 : hdlBasic/Constant  const=r  gui_display_data_type=Fixed-point  arith_type=Unsigned  n_bits=n  bin_pt=0  preci_type=Single  exp_width=8  frac_width=24  explicit_period=off  period=1  XmcBlockStatus=1  maskContainerNames=tabcontainer1  block_type=constant  block_config=sysgen:Constant_config
  Mux : hdlBasic/Mux  inputs=2  en=off  latency=0  precision=Full  arith_type=Unsigned  n_bits=16  bin_pt=14  quantization=Truncate  overflow=Wrap  XmcBlockStatus=1  maskContainerNames=tabcontainer1  block_type=mux  block_config=sysgen:Mux_config
  Register : hdlBasic/Register  init=0  rst=off  en=off  XmcBlockStatus=1  maskContainerNames=tabcontainer1  block_type=register  block_config=sysgen:Register_config
  Relational : hdlBasic/Relational  mode=a>b  op_type=Bool  en=off  latency=0  XmcBlockStatus=1  maskContainerNames=tabcontainer1  block_type=relational  block_config=sysgen:Relational_config
  Relational1 : hdlBasic/Relational  mode=a>b  op_type=Bool  en=off  latency=0  XmcBlockStatus=1  maskContainerNames=tabcontainer1  block_type=relational  block_config=sysgen:Relational_config
  Strobe : Outport  VectorParamsAs1DForOutWhenUnconnected=off
  wires:
  Mux/1 -> AddSub/1
  Relational1/1 -> Mux/1
  AddSub2/1 -> Mux/3
  Constant1/1 -> Relational1/2, AddSub2/2
  Register/1 -> Relational/1, Relational1/1, Mux/2, AddSub2/1
  AddSub/1 -> Register/1, Relational/2
  Relational/1 -> Strobe/1
  Error/1 -> AddSub1/2
  Constant/1 -> AddSub1/1
  AddSub1/1 -> AddSub/2

== system demonstrator/Receiver/Time Synchronisation/Timing Error Detector ==
  Real In : Inport
  Imag In : Inport  Port=2
  AddSub : hdlBasic/AddSub  mode=Subtraction  use_carryin=off  use_carryout=off  en=off  latency=0  precision=User Defined  arith_type="Signed  (2's comp)"  n_bits=31  bin_pt=30  quantization=Truncate  overflow=Saturate  use_behavioral_HDL=off  hw_selection=Fabric  pipelined=off  XmcBlockStatus=1  maskContainerNames=tabcontainer1  block_type=addsub  block_config=sysgen:Addsub_config
  AddSub1 : hdlBasic/AddSub  mode=Subtraction  use_carryin=off  use_carryout=off  en=off  latency=0  precision=User Defined  arith_type="Signed  (2's comp)"  n_bits=31  bin_pt=30  quantization=Truncate  overflow=Saturate  use_behavioral_HDL=off  hw_selection=Fabric  pipelined=off  XmcBlockStatus=1  maskContainerNames=tabcontainer1  block_type=addsub  block_config=sysgen:Addsub_config
  AddSub2 : hdlBasic/AddSub  mode=Addition  use_carryin=off  use_carryout=off  en=off  latency=0  precision=Full  arith_type="Signed  (2's comp)"  n_bits=16  bin_pt=13  quantization="Round  (unbiased: +/- Inf)"  overflow=Saturate  use_behavioral_HDL=off  hw_selection=Fabric  pipelined=off  XmcBlockStatus=1  maskContainerNames=tabcontainer1  block_type=addsub  block_config=sysgen:Addsub_config
  CMult : hdlBasic/CMult  const=10  gui_display_data_type=Fixed-point  const_n_bits=4  const_bin_pt=0  float_type=Single  exp_bits=8  fraction_bits=24  en=off  latency=0  precision=User Defined  arith_type="Signed  (2's comp)"  n_bits=32  bin_pt=30  quantization=Truncate  overflow=Saturate  use_behavioral_HDL=off  mem_type=Distributed RAM  pipeline=off  XmcBlockStatus=1  maskContainerNames=tabcontainer1  block_type=cmult  block_config=sysgen:CMult_config
      settings: infoedit=[]
  Delay : hdlBasic/Delay  rst=off  en=off  latency=32  reg_retiming=off  XmcBlockStatus=1  maskContainerNames=group1  block_type=delay  block_config=sysgen:Delay_config
  Delay1 : hdlBasic/Delay  rst=off  en=off  latency=32  reg_retiming=off  XmcBlockStatus=1  maskContainerNames=group1  block_type=delay  block_config=sysgen:Delay_config
  Mult1 : hdlBasic/Mult  precision=User Defined  arith_type=Unsigned  n_bits=31  bin_pt=30  quantization=Truncate  overflow=Saturate  en=off  latency=0  use_behavioral_HDL=off  opt=Speed  use_embedded=on  optimum_pipeline=off  pipeline=on  use_rpm=on  placement_style=Triangular  XmcBlockStatus=1  maskContainerNames=group1  block_type=mult  block_config=sysgen:Mult_config
  Mult2 : hdlBasic/Mult  precision=User Defined  arith_type=Unsigned  n_bits=31  bin_pt=30  quantization=Truncate  overflow=Saturate  en=off  latency=0  use_behavioral_HDL=off  opt=Speed  use_embedded=on  optimum_pipeline=off  pipeline=on  use_rpm=on  placement_style=Triangular  XmcBlockStatus=1  maskContainerNames=group1  block_type=mult  block_config=sysgen:Mult_config
  Reinterpret : hdlBasic/Reinterpret  force_arith_type=on  arith_type="Signed  (2's comp)"  force_bin_pt=on  bin_pt=15  XmcBlockStatus=1  maskContainerNames=group1  block_type=reinterpret  block_config=sysgen:Reinterpret_config
  Reinterpret1 : hdlBasic/Reinterpret  force_arith_type=on  arith_type="Signed  (2's comp)"  force_bin_pt=on  bin_pt=15  XmcBlockStatus=1  maskContainerNames=group1  block_type=reinterpret  block_config=sysgen:Reinterpret_config
  Error : Outport  VectorParamsAs1DForOutWhenUnconnected=off
  wires:
  Reinterpret1/1 -> Mult1/2, Mult1/1
  Reinterpret/1 -> Mult2/1, Mult2/2
  Delay/1 -> AddSub/2
  Mult1/1 -> Delay/1, AddSub/1
  AddSub1/1 -> AddSub2/2
  Mult2/1 -> AddSub1/1, Delay1/1
  Delay1/1 -> AddSub1/2
  AddSub2/1 -> CMult/1
  AddSub/1 -> AddSub2/1
  Imag In/1 -> Reinterpret/1
  Real In/1 -> Reinterpret1/1
  CMult/1 -> Error/1
